simulink model "dbsim"  (R2024b)
settings: Solver=VariableStepAuto  StartTime=0.0  StopTime=20  RelTol=1e-3
values from neighbouring files (symbols this model uses):
  dirsorder = [11 12]    [main.m]
  dtflin = dtftust(tflin, Ts)    [disc.m]    (also in main.m)
  tfDBReg = DBReg(dtflin)    [main.m]
  z = -0.1    [main.m]
settings Model: Creator=markminerov  LastModifiedBy=markminerov
settings DebuggingCC: AlgebraicLoopMsg=none

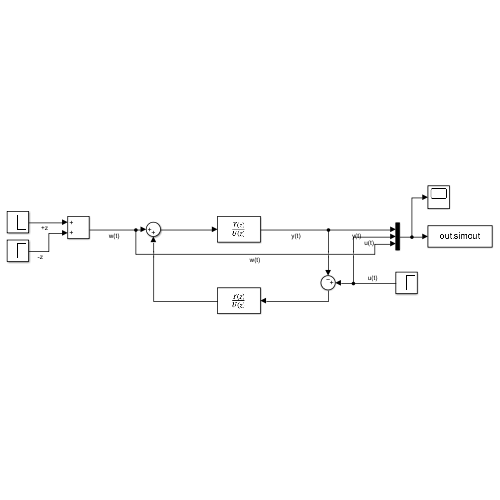
[thumbnail: Simulink's stored preview of the top-level diagram]
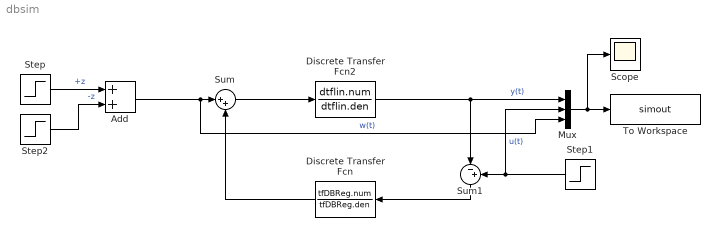
== system dbsim ==
  Add : Sum
  Discrete Transfer Fcn : DiscreteTransferFcn  Numerator=tfDBReg.num  Denominator=tfDBReg.den
  Discrete Transfer Fcn2 : DiscreteTransferFcn  Numerator=dtflin.num  Denominator=dtflin.den
  Mux : Mux  Inputs=3
  Scope : Scope
  Step : Step  Time=dirsorder(1)  After=z  SampleTime=0
  Step1 : Step  After=u  SampleTime=0
  Step2 : Step  Time=dirsorder(2)  After=-z  SampleTime=0
  Sum : Sum  Inputs=|++
  Sum1 : Sum  Inputs=|-+
  To Workspace : ToWorkspace  VariableName=simout  SaveFormat=Timeseries  SampleTime=-1
  wires:
  Discrete Transfer Fcn/1 -> Sum/2
  Discrete Transfer Fcn2/1 -> Sum1/1, Mux/1  "y(t)"
  Sum/1 -> Discrete Transfer Fcn2/1
  Step/1 -> Add/1  "+z"
  Step2/1 -> Add/2  "-z"
  Add/1 -> Mux/3, Sum/1  "w(t)"
  Sum1/1 -> Discrete Transfer Fcn/1
  Step1/1 -> Mux/2, Sum1/2  "u(t)"
  Mux/1 -> Scope/1, To Workspace/1
